simulink model "Q6_b_second_solution"  (R2017a)
settings: Solver=FixedStepAuto  StartTime=0.0  StopTime=10.0  FixedStep=0.01  RelTol=0.00001
model workspace (MAT data in the model file):
  Kp_1 = 10000
  Kp_2 = 10000
  Kv_1 = 200
  Kv_2 = 200
  a_1 = 1
  a_2 = 1
  g = 9.8
  m_1 = 1
  m_2 = 1
  theta_d_dot = 1
  theta_d_double_dot = 1
libraries: simulink x5
settings Model: Creator=Omer  LastModifiedBy=Omer
settings ModelReferenceCC: ModelReferenceMinAlgLoopOccurrences=on

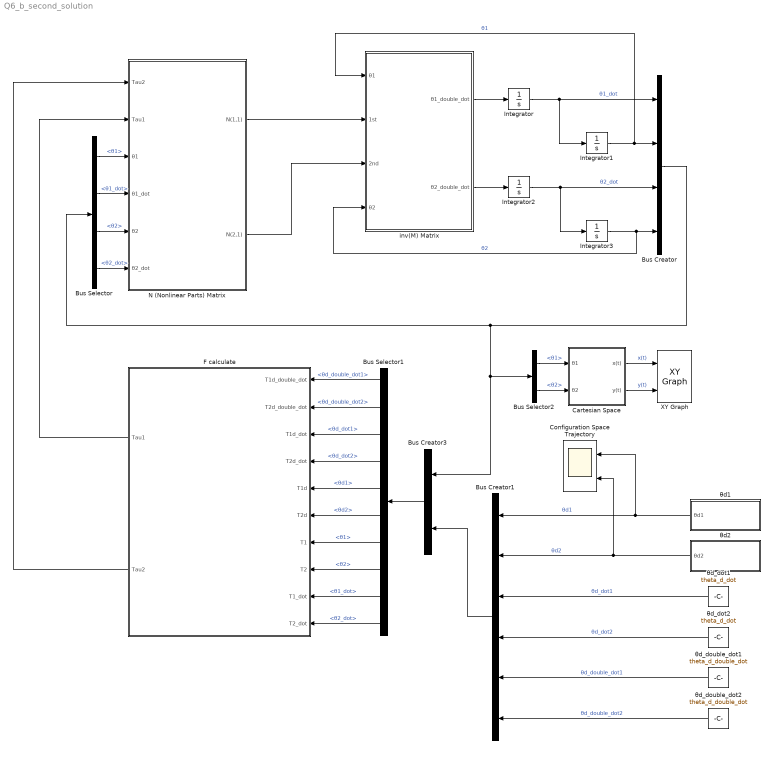
== system Q6_b_second_solution ==
  Bus Creator : BusCreator  Inputs=4
  Bus Creator1 : BusCreator  Inputs=6
  Bus Creator3 : BusCreator  Inputs=2
  Bus Selector : BusSelector  OutputSignals=θ1,θ1_dot,θ2,θ2_dot
  Bus Selector1 : BusSelector  OutputSignals=signal2.θd_double_dot1,signal2.θd_double_dot2,signal2.θd_dot1,signal2.θd_dot2,signal2.θd1,signal2.θd2,signal1.θ1,signal1.θ2,signal1.θ1_dot,signal1.θ2_dot
  Bus Selector2 : BusSelector  OutputSignals=θ1,θ2
  "Cartesian Space " : Subsystem  TreatAsAtomicUnit=on
  Configuration Space Trajectory : Scope  NumInputPorts=2
  F calculate : MATLAB Function  TreatAsAtomicUnit=on
  Integrator{,1..3} (4 alike) : Integrator
  N (Nonlinear Parts) Matrix : Subsystem  TreatAsAtomicUnit=on
  XY Graph : simulink/Sinks/XY Graph  xmin=-1  xmax=3  ymin=-1  ymax=2  st=-1
  inv(M) Matrix : Subsystem  TreatAsAtomicUnit=on
  θd1 : Subsystem  TreatAsAtomicUnit=on
  θd2 : Subsystem  TreatAsAtomicUnit=on
  θd_dot1 : Constant  Value=theta_d_dot
  θd_dot2 : Constant  Value=theta_d_dot
  θd_double_dot1 : Constant  Value=theta_d_double_dot
  θd_double_dot2 : Constant  Value=theta_d_double_dot
  wires:
  N (Nonlinear Parts) Matrix/2(N(2,1)) -> inv(M) Matrix/3(2nd)
  N (Nonlinear Parts) Matrix/1(N(1,1)) -> inv(M) Matrix/2(1st)
  Bus Creator/1 -> Bus Creator3/1, Bus Selector2/1, Bus Selector/1
  inv(M) Matrix/2(θ2_double_dot) -> Integrator2/1
  Bus Selector/1 -> N (Nonlinear Parts) Matrix/3("θ1 ")  "<θ1>"
  Integrator2/1 -> Integrator3/1, Bus Creator/3  "θ2_dot"
  Integrator3/1 -> inv(M) Matrix/4(θ2), Bus Creator/4  "θ2"
  Integrator1/1 -> inv(M) Matrix/1(θ1), Bus Creator/2  "θ1"
  Bus Selector/3 -> N (Nonlinear Parts) Matrix/5(θ2)  "<θ2>"
  Bus Selector/2 -> N (Nonlinear Parts) Matrix/4(θ1_dot)  "<θ1_dot>"
  Integrator/1 -> Bus Creator/1, Integrator1/1  "θ1_dot"
  Bus Selector/4 -> N (Nonlinear Parts) Matrix/6(θ2_dot)  "<θ2_dot>"
  inv(M) Matrix/1(θ1_double_dot) -> Integrator/1
  Bus Selector2/1 -> "Cartesian Space "/1(θ1)  "<θ1>"
  Bus Selector2/2 -> "Cartesian Space "/2(θ2)  "<θ2>"
  "Cartesian Space "/1(x(t)) -> XY Graph/1  "x(t)"
  "Cartesian Space "/2(y(t)) -> XY Graph/2  "y(t)"
  Bus Creator1/1 -> Bus Creator3/2
  θd_dot1/1 -> Bus Creator1/3  "θd_dot1"
  θd_dot2/1 -> Bus Creator1/4  "θd_dot2"
  θd_double_dot1/1 -> Bus Creator1/5  "θd_double_dot1"
  θd_double_dot2/1 -> Bus Creator1/6  "θd_double_dot2"
  θd1/1(θd1) -> Configuration Space Trajectory/1, Bus Creator1/1  "θd1"
  θd2/1(θd2) -> Bus Creator1/2, Configuration Space Trajectory/2  "θd2"
  F calculate/2(Tau2) -> N (Nonlinear Parts) Matrix/1(Tau2)
  F calculate/1(Tau1) -> N (Nonlinear Parts) Matrix/2(Tau1)
  Bus Selector1/2 -> F calculate/2(T2d_double_dot)  "<θd_double_dot2>"
  Bus Selector1/9 -> F calculate/9(T1_dot)  "<θ1_dot>"
  Bus Selector1/1 -> F calculate/1(T1d_double_dot)  "<θd_double_dot1>"
  Bus Selector1/8 -> F calculate/8(T2)  "<θ2>"
  Bus Selector1/5 -> F calculate/5(T1d)  "<θd1>"
  Bus Selector1/7 -> F calculate/7(T1)  "<θ1>"
  Bus Selector1/10 -> F calculate/10(T2_dot)  "<θ2_dot>"
  Bus Selector1/4 -> F calculate/4(T2d_dot)  "<θd_dot2>"
  Bus Selector1/3 -> F calculate/3(T1d_dot)  "<θd_dot1>"
  Bus Selector1/6 -> F calculate/6(T2d)  "<θd2>"
  Bus Creator3/1 -> Bus Selector1/1

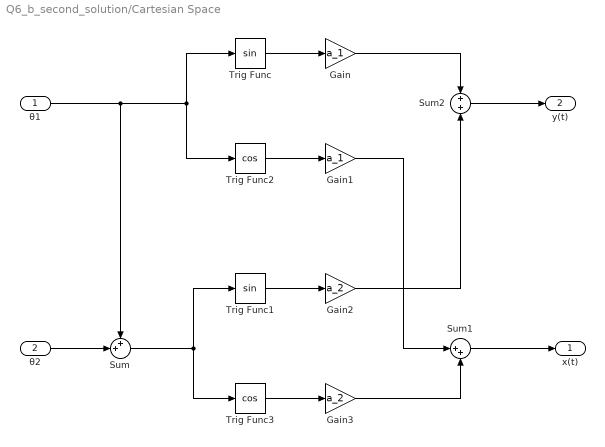
== system Q6_b_second_solution/Cartesian Space  ==
  θ1 : Inport
  θ2 : Inport  Port=2
  Gain : Gain  Gain=a_1
  Gain1 : Gain  Gain=a_1
  Gain2 : Gain  Gain=a_2
  Gain3 : Gain  Gain=a_2
  Sum : Sum  Inputs=++|
  Sum1 : Sum  Inputs=|++
  Sum2 : Sum  Inputs=+|+
  Trig Func : Trigonometry
  Trig Func1 : Trigonometry
  Trig Func2 : Trigonometry  Operator=cos
  Trig Func3 : Trigonometry  Operator=cos
  x(t) : Outport
  y(t) : Outport  Port=2
  wires:
  θ1/1 -> Trig Func2/1, Trig Func/1, Sum/1
  θ2/1 -> Sum/2
  Sum/1 -> Trig Func3/1, Trig Func1/1
  Sum2/1 -> y(t)/1
  Sum1/1 -> x(t)/1
  Trig Func/1 -> Gain/1
  Gain/1 -> Sum2/1
  Trig Func2/1 -> Gain1/1
  Gain1/1 -> Sum1/1
  Trig Func1/1 -> Gain2/1
  Gain2/1 -> Sum2/2
  Trig Func3/1 -> Gain3/1
  Gain3/1 -> Sum1/2

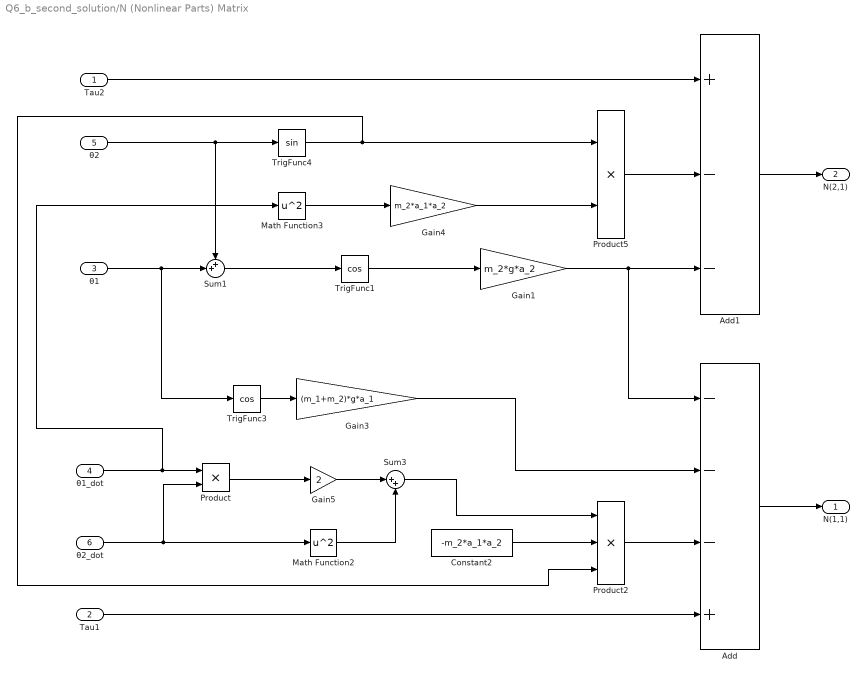
== system Q6_b_second_solution/N (Nonlinear Parts) Matrix ==
  Tau2 : Inport
  Tau1 : Inport  Port=2
  "θ1 " : Inport  Port=3
  θ1_dot : Inport  Port=4
  θ2 : Inport  Port=5
  θ2_dot : Inport  Port=6
  Add : Sum  Inputs=---+
  Add1 : Sum  Inputs=+--
  Constant2 : Constant  Value=-m_2*a_1*a_2
  Gain1 : Gain  Gain=m_2*g*a_2
  Gain3 : Gain  Gain=(m_1+m_2)*g*a_1
  Gain4 : Gain  Gain=m_2*a_1*a_2
  Gain5 : Gain  Gain=2
  Math Function2 : Math  Operator=square  SaturateOnIntegerOverflow=on
  Math Function3 : Math  Operator=square  SaturateOnIntegerOverflow=on
  Product : Product
  Product2 : Product  Inputs=3
  Product5 : Product
  Sum1 : Sum  Inputs=++|
  Sum3 : Sum  Inputs=|++
  TrigFunc1 : Trigonometry  Operator=cos
  TrigFunc3 : Trigonometry  Operator=cos
  TrigFunc4 : Trigonometry
  N(1,1) : Outport
  N(2,1) : Outport  Port=2
  wires:
  Product2/1 -> Add/3
  Gain3/1 -> Add/2
  θ2/1 -> TrigFunc4/1, Sum1/1
  TrigFunc4/1 -> Product2/3, Product5/1
  Add1/1 -> N(2,1)/1
  Math Function3/1 -> Gain4/1
  θ1_dot/1 -> Product/1, Math Function3/1
  θ2_dot/1 -> Product/2, Math Function2/1
  Sum1/1 -> TrigFunc1/1
  Add/1 -> N(1,1)/1
  Sum3/1 -> Product2/1
  Math Function2/1 -> Sum3/2
  Tau2/1 -> Add1/1
  Constant2/1 -> Product2/2
  TrigFunc3/1 -> Gain3/1
  TrigFunc1/1 -> Gain1/1
  "θ1 "/1 -> TrigFunc3/1, Sum1/2
  Product5/1 -> Add1/2
  Tau1/1 -> Add/4
  Gain4/1 -> Product5/2
  Gain1/1 -> Add1/3, Add/1
  Product/1 -> Gain5/1
  Gain5/1 -> Sum3/1

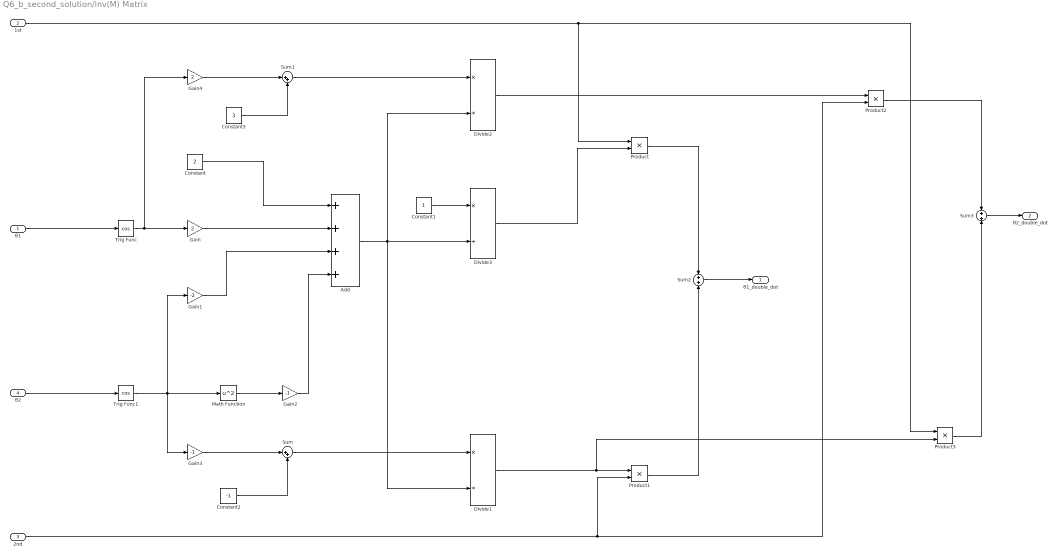
== system Q6_b_second_solution/inv(M) Matrix ==
  θ1 : Inport
  1st : Inport  Port=2
  2nd : Inport  Port=3
  θ2 : Inport  Port=4
  Add : Sum  Inputs=4
  Constant : Constant  Value=2
  Constant1 : Constant
  Constant2 : Constant  Value=-1
  Constant3 : Constant  Value=3
  Divide1 : Product  Inputs=*/
  Divide2 : Product  Inputs=*/
  Divide3 : Product  Inputs=*/
  Gain : Gain  Gain=2
  Gain1 : Gain  Gain=-2
  Gain2 : Gain  Gain=-1
  Gain3 : Gain  Gain=-1
  Gain4 : Gain  Gain=2
  Math Function : Math  Operator=square  SaturateOnIntegerOverflow=on
  Product{,1..3} (4 alike) : Product
  Sum : Sum  Inputs=|++
  Sum1 : Sum  Inputs=|++
  Sum2 : Sum  Inputs=+|+
  Sum3 : Sum  Inputs=+|+
  Trig Func : Trigonometry  Operator=cos
  Trig Func1 : Trigonometry  Operator=cos
  θ1_double_dot : Outport
  θ2_double_dot : Outport  Port=2
  wires:
  Add/1 -> Divide2/2, Divide3/2, Divide1/2
  θ1/1 -> Trig Func/1
  θ2/1 -> Trig Func1/1
  Trig Func1/1 -> Gain3/1, Gain1/1, Math Function/1
  Trig Func/1 -> Gain4/1, Gain/1
  Constant/1 -> Add/1
  Gain/1 -> Add/2
  Gain1/1 -> Add/3
  Constant1/1 -> Divide3/1
  Math Function/1 -> Gain2/1
  Gain2/1 -> Add/4
  Gain3/1 -> Sum/1
  Constant2/1 -> Sum/2
  Sum/1 -> Divide1/1
  Constant3/1 -> Sum1/2
  Gain4/1 -> Sum1/1
  1st/1 -> Product/1, Product3/1
  Divide3/1 -> Product/2
  Divide1/1 -> Product3/2, Product1/1
  2nd/1 -> Product2/2, Product1/2
  Product/1 -> Sum2/1
  Product1/1 -> Sum2/2
  Sum2/1 -> θ1_double_dot/1
  Sum1/1 -> Divide2/1
  Divide2/1 -> Product2/1
  Product2/1 -> Sum3/1
  Sum3/1 -> θ2_double_dot/1
  Product3/1 -> Sum3/2

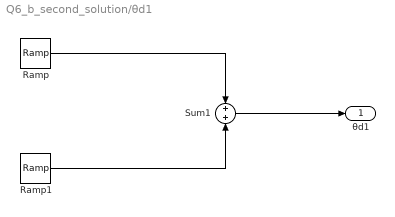
== system Q6_b_second_solution/θd1 ==
  Ramp : simulink/Sources/Ramp  slope=pi/12  start=0  X0=0
  Ramp1 : simulink/Sources/Ramp  slope=-pi/12  start=2  X0=0
  Sum1 : Sum  Inputs=+|+
  θd1 : Outport
  wires:
  Sum1/1 -> θd1/1
  Ramp/1 -> Sum1/1
  Ramp1/1 -> Sum1/2

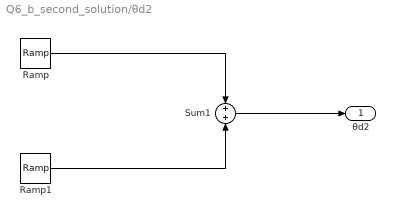
== system Q6_b_second_solution/θd2 ==
  Ramp : simulink/Sources/Ramp  slope=pi/3  start=0  X0=0
  Ramp1 : simulink/Sources/Ramp  slope=-pi/3  start=2  X0=0
  Sum1 : Sum  Inputs=+|+
  θd2 : Outport
  wires:
  Sum1/1 -> θd2/1
  Ramp/1 -> Sum1/1
  Ramp1/1 -> Sum1/2

== matlab function Q6_b_second_solution/F calculate ==
  data: T1d_double_dot input; T2d_double_dot input; T1d_dot input; T2d_dot input; T1d input; T2d input; Tau1 output; T1 input; T2 input; T1_dot input; T2_dot input; Tau2 output
function [Tau1, Tau2] = fcn(T1d_double_dot, T2d_double_dot, T1d_dot, T2d_dot, T1d, T2d, T1, T2, T1_dot, T2_dot)
Kv = 200; Kp = 10000; g = 9.8;

e = zeros(2,1);
e_dot = zeros(2,1);
e = [T1d - T1; T2d - T2];
e_dot = [T1d_dot - T1_dot; T2d_dot - T2_dot];

M = @(T2) [3+2*cos(T2) 1+cos(T2); 1+cos(T2) 1];
N = @(T1,T2,T1_dot,T2_dot) [-(2*T1_dot*T2_dot+T2_dot^2)*sin(T2) + 2*g*cos(T1) + g*cos(T1+T2);
     T1_dot^2*sin(T2) + g*cos(T1+T2)];

Tau = M(T2)*(T1d_double_dot + [Kv 0; 0 Kv]*e_dot + [Kp 0; 0 Kp]*e) + N(T1,T2,T1_dot,T2_dot);
Tau1 = Tau(1,1);
Tau2 = Tau(2,1);
